simulink model "SimplePropellerModel_Soln"  (R2025a)
settings: Solver=VariableStepAuto  StartTime=0.0  StopTime=10.0  RelTol=1e-3
undefined symbols (not defined in the file): km, kT, magnitude
settings Model: Creator=esmithzb  LastModifiedBy=esmithzb
settings DebuggingCC: UnderspecifiedInitializationDetection=Classic  MergeDetectMultiDrivingBlocksExec=none
settings ModelReferenceCC: PropagateSignalLabelsOutOfModel=off
settings SimscapeCC: SimscapeNominalValues="[{\"value\":\"1\",\"unit\":\"A\"},{\"value\":\"1\",\"unit\":\"bar\"},{\"value\":\"1\",\"unit\":\"cm^2\"},{\"value\":\"1\",\"unit\":\"cm^3/s\"},{\"value\":\"1\",\"unit\":\"kJ/kg\"},{\"value\":\"1\",\"unit\":\"kW\"},{\"value\":\"1\",\"unit\":\"l\"},{\"value\":\"1\",\"unit\":\"N\"},{\"value\":\"1\",\"unit\":\"N*m\"},{\"value\":\"1\",\"unit\":\"V\"},{\"value\":\"0.001\",\"unit\":\"Wb\"}]"  SimscapeLogType=all  SimscapeLogDataHistory=10000.0

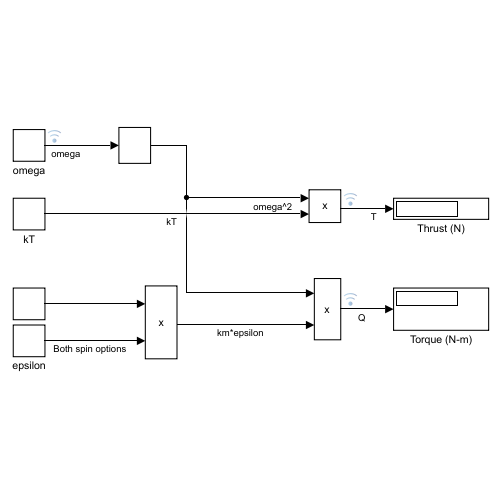
[thumbnail: Simulink's stored preview of the top-level diagram]
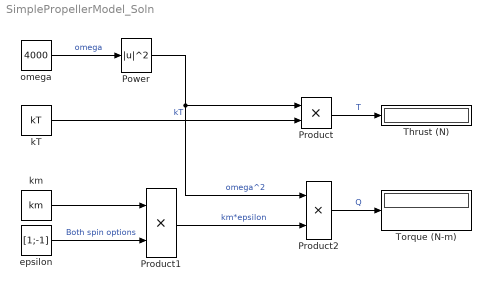
== system SimplePropellerModel_Soln ==
  Power : Math  Operator=magnitude^2
  Product : Product
  Product1 : Product
  Product2 : Product
  Thrust (N) : Display
  Torque (N-m) : Display
  epsilon : Constant  Value=[1;-1]
  kT : Constant  Value=kT
  km : Constant  Value=km
  omega : Constant  Value=4000
  wires:
  Power/1 -> Product2/1, Product/1  "omega^2"
  kT/1 -> Product/2  "kT"
  Product/1 -> Thrust (N)/1  "T"
  km/1 -> Product1/1
  Product2/1 -> Torque (N-m)/1  "Q"
  Product1/1 -> Product2/2  "km*epsilon"
  omega/1 -> Power/1  "omega"
  epsilon/1 -> Product1/2  "Both spin options"
